simulink model "PSM3_Information_Penkov_Nikolay_Testframework_Gesamtsystem"  (R2012b)
settings: Solver=FixedStepDiscrete  StartTime=0.0  StopTime=320  FixedStep=0.00001  RelTol=1e-3
libraries: idelinklib_tgtpref x1
settings Model: Creator=Nikolay  LastModifiedBy=Nikolay
settings DataIOCC: SaveOutput=off  SaveTime=off
settings OptimizationCC: OptimizeModelRefInitCode=on  LifeSpan=1
settings HardwareCC: ProdBitPerChar=16  ProdBitPerInt=16  ProdBitPerPointer=16  ProdLargestAtomicInteger=Integer  ProdIntDivRoundTo=Zero  ProdEndianess=LittleEndian  ProdWordSize=16  ProdHWDeviceType=Texas Instruments->C2000
settings RTWCC: SystemTargetFile=idelink_ert.tlc  GenerateMakefile=off  TemplateMakefile=none  Description=IDE Link ERT  ProcessScript=idelink_ert_make_rtw_hook
settings CodeAppCC: IgnoreCustomStorageClasses=off

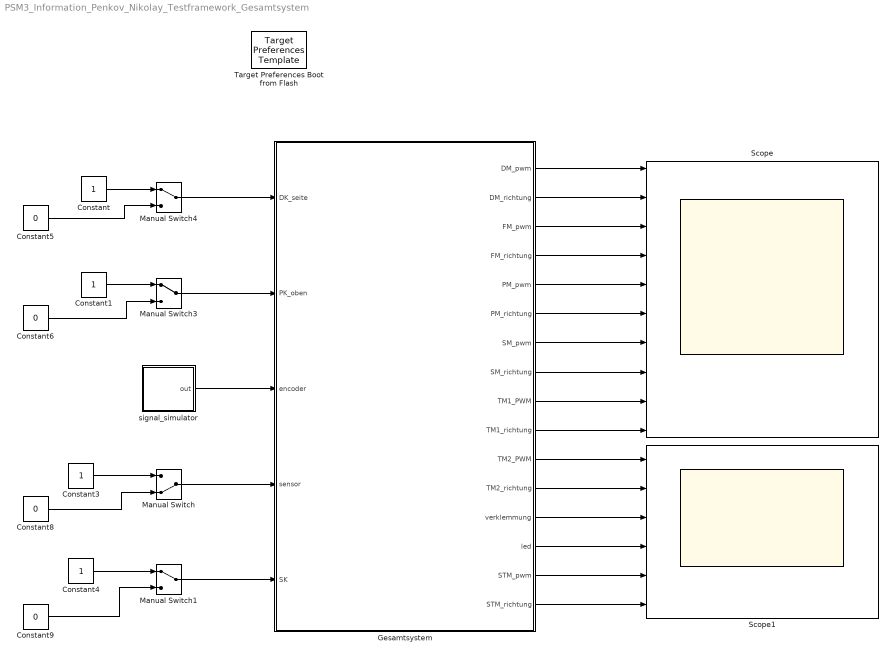
== system PSM3_Information_Penkov_Nikolay_Testframework_Gesamtsystem ==
  Constant{,1,3..4} (4 alike) : Constant
  Constant{5..6,8..9} (4 alike) : Constant  Value=0
  Gesamtsystem : Stateflow chart  TreatAsAtomicUnit=on
  Manual Switch : ManualSwitch  CurrentSetting=0
  Manual Switch1 : ManualSwitch
  Manual Switch3 : ManualSwitch
  Manual Switch4 : ManualSwitch
  Scope : Scope  NumInputPorts=10
      settings: ShowLegends=on  YMin=-1~-1~0~-5~0~-5~-5~-5~-5~-5  YMax=1~1~75~5~100~5~5~5~5~5
  Scope1 : Scope  NumInputPorts=6
      settings: YMin=-5~-5~-5~-5~57~-5  YMax=5~5~5~5~63~5
  Target Preferences Boot from Flash : idelinklib_tgtpref/Target Preferences Template  Tag=ccslinktgtpref_ccsv4  library=off
  signal_simulator : Stateflow chart  TreatAsAtomicUnit=on
  wires:
  signal_simulator/1(out) -> Gesamtsystem/3(encoder)
  Manual Switch1/1 -> Gesamtsystem/5(SK)
  Manual Switch/1 -> Gesamtsystem/4(sensor)
  Manual Switch3/1 -> Gesamtsystem/2(PK_oben)
  Manual Switch4/1 -> Gesamtsystem/1(DK_seite)
  Constant/1 -> Manual Switch4/1
  Constant1/1 -> Manual Switch3/1
  Constant3/1 -> Manual Switch/1
  Constant4/1 -> Manual Switch1/1
  Constant5/1 -> Manual Switch4/2
  Constant6/1 -> Manual Switch3/2
  Constant8/1 -> Manual Switch/2
  Constant9/1 -> Manual Switch1/2
  Gesamtsystem/1(DM_pwm) -> Scope/1
  Gesamtsystem/2(DM_richtung) -> Scope/2
  Gesamtsystem/3(FM_pwm) -> Scope/3
  Gesamtsystem/4(FM_richtung) -> Scope/4
  Gesamtsystem/5(PM_pwm) -> Scope/5
  Gesamtsystem/6(PM_richtung) -> Scope/6
  Gesamtsystem/7(SM_pwm) -> Scope/7
  Gesamtsystem/8(SM_richtung) -> Scope/8
  Gesamtsystem/9(TM1_PWM) -> Scope/9
  Gesamtsystem/10(TM1_richtung) -> Scope/10
  Gesamtsystem/11(TM2_PWM) -> Scope1/1
  Gesamtsystem/12(TM2_richtung) -> Scope1/2
  Gesamtsystem/13(verklemmung) -> Scope1/3
  Gesamtsystem/14(led) -> Scope1/4
  Gesamtsystem/15(STM_pwm) -> Scope1/5
  Gesamtsystem/16(STM_richtung) -> Scope1/6

== stateflow chart PSM3_Information_Penkov_Nikolay_Testframework_Gesamtsystem/Gesamtsystem ==
  state Motor_Foerderbahn_Check [parallel]
    settings: executionOrder=3
    state Start
    state Encoder_abfrage
      zustand_vor = encoder;
    state Naechster_Wert
      zustand_nach = encoder;
    state Vergleich
      vrgl = zustand_nach - zustand_vor;
    state Verklemmt
      verklemmung = true;
    state Nicht_Verklemmt
      verklemmung = false;
    (default) -> Motor_Foerderbahn_Check.Start
    Verklemmt -> Motor_Foerderbahn_Check.Start
    Nicht_Verklemmt -> Motor_Foerderbahn_Check.Start
    Motor_Foerderbahn_Check.Start -> Encoder_abfrage
    Encoder_abfrage -> Naechster_Wert : [after(3,sec)]
    Naechster_Wert -> Vergleich
    Vergleich -> Nicht_Verklemmt [order 2] : [abs(vrgl) == 1]
    Vergleich -> Verklemmt [order 1] : [abs(vrgl) == 0]
  state Teilsystem_1 [parallel]
    settings: executionOrder=1
    state Start
      c = 0;
      turm1_gebaut  = false;
      turm2_gebaut = false;
      led = false;
    state Foerderbahn_start
      en: FM_pwm = 60;
      FM_richtung = 0;
    state System_idle
      FM_pwm = 0;
      TS1_aktivate = false;
      TS2_aktivate = true;
    (default) -> Teilsystem_1.Start
    Teilsystem_1.Start -> Foerderbahn_start
    Teilsystem_1.System_idle -> Foerderbahn_start : [TS1_aktivate == true]
    Foerderbahn_start -> Teilsystem_1.System_idle : [sensor == 0]
  note: INFO: FM_richtung
      | 0 - nach vorne
      | 1 - nach hinten
  state Teilsystem_2 [parallel]
    settings: executionOrder=4
    state TS1_freigabe
      TS2_aktivate = false;
      TS1_aktivate = true;
    state Start
    state Fertig
      led = 1;
    state Platforme_hoch_1
      PM_richtung = 0;
      PM_pwm = 100;
    state System_idle
      TS2_aktivate = false;
      TS3_aktivate = true;
      PM_pwm = 0;
      ex: c = 0;
    state Increment_und_check
      c = c + 1;
    state Plattforme_mittelstop
      PM_pwm = 0;
    state Platforme_runter
      SM_pwm = 0;
      PM_richtung = 1;
      PM_pwm = 100;
    state Stab_entfernen
      STM_richtung = 0;
      STM_pwm = 60;
    state Stab_setzen
      PM_pwm = 0;
      STM_richtung = 1;
      STM_pwm = 60;
    state Platforme_hoch_2
      STM_pwm = 0;
      PM_pwm = 100;
    (default) -> Teilsystem_2.Start
    TS1_freigabe -> Teilsystem_2.Start
    Teilsystem_2.System_idle -> TS1_freigabe [order 1] : [turm2_gebaut == false && TS2_aktivate == true]
    Teilsystem_2.Start -> Platforme_hoch_1 : [TS2_aktivate == true]
    Increment_und_check -> TS1_freigabe [order 2] : [c < 6]
    (junction 437) -> TS1_freigabe [order 2] : [c < 9 && turm1_gebaut == true]
    Teilsystem_2.System_idle -> Fertig [order 2] : [turm2_gebaut == true && TS2_aktivate == true ]
    Platforme_hoch_1 -> Plattforme_mittelstop : after(300,tick)
    (junction 437) -> Teilsystem_2.System_idle [order 1] : [turm1_gebaut == false && c == 6]
    (junction 437) -> Teilsystem_2.System_idle [order 3] : [turm1_gebaut == true && c == 9]
    Increment_und_check -> (junction 437) [order 1] : [c >= 6]
    Plattforme_mittelstop -> Stab_entfernen
    Platforme_runter -> Increment_und_check : after(2,sec)
    Stab_entfernen -> Platforme_hoch_2 : [SK == true]
    Stab_setzen -> Platforme_runter : after(2,sec)
    Platforme_hoch_2 -> Stab_setzen : after(2,sec)
  state Teilsystem_3 [parallel]
    settings: executionOrder=2
    state TS2_freigabe
      TS3_aktivate = false;
      TS2_aktivate = true;
      c =0;
    state Motoren_unter
      TM1_richtung = 1;
      TM2_richtung = 1;
      TM1_PWM = 100;
      TM2_PWM = 100;
      DM_pwm = 0;
    state Start
    state Magazin_transport
      TM1_richtung = 0;
      TM2_richtung = 0;
      TM1_PWM = 100;
      TM2_PWM = 100;
    state Drehen_zureuck
      SM_pwm = 0;
      DM_richtung = 1;
      DM_pwm = 60;
    state Schieber_zureuck
      TM1_PWM = 0;
      TM2_PWM = 0;
      SM_richtung = 1;
      SM_pwm = 60;
    state Hohe_abfrage
      TM1_PWM = 0;
      TM2_PWM = 0;
    state Turm_befreien
      TM1_PWM = 100;
      TM2_PWM = 100;
    state Drehen_T1
      DM_pwm = 60;
      DM_richtung = 0;
      turm1_gebaut = true;
    state Schieber_warten
      SM_pwm = 0;
    state Schieber_fahren
      DM_pwm =0
      SM_richtung = 0;
      SM_pwm = 60;
    state Drehen_T2
      DM_pwm = 60;
      DM_richtung = 0;
      turm2_gebaut = true;
    (default) -> Teilsystem_3.Start
    TS2_freigabe -> Teilsystem_3.Start
    Motoren_unter -> TS2_freigabe : after(3,sec)
    Teilsystem_3.Start -> Magazin_transport : [TS3_aktivate == true]
    Drehen_zureuck -> Motoren_unter : [DK_seite == true]
    Magazin_transport -> Hohe_abfrage : after(3,sec)
    Schieber_zureuck -> Drehen_zureuck : after(1,sec)
    Hohe_abfrage -> (junction 262)
    Turm_befreien -> Schieber_zureuck : after(5,sec)
    Schieber_warten -> Turm_befreien : after(1,sec)
    (junction 262) -> Drehen_T1 [order 1] : [turm1_gebaut == false]
    (junction 262) -> Drehen_T2 [order 2] : [turm1_gebaut == true && turm2_gebaut == false]
    Drehen_T1 -> Schieber_fahren : after(2,sec)
    Schieber_fahren -> Schieber_warten : after(1,sec)
    Drehen_T2 -> Schieber_fahren : after(4,sec)
  note: INFO: PM_richtung
      | 0 - nach oben
      | 1 - nach unten
  note: INFO: TM_richtung
      | 0 - nach oben
      | 1 - nach unten
  note: INFO: STM_richtung
      | 0 - nach hinten
      | 1 - nach vorne
  note: INFO: SM_richtung
      | 0 - nach vorne
      | 1 - nach hinten
  note: INFO: DM_richtung
      | 0 - gegen den Uhrzeigersinn
      | 1 - im Uhrzeigersinn
  data: DK_seite input; PK_oben input; encoder input; sensor input; turm2_gebaut local double; DM_pwm output double; DM_richtung output double; FM_pwm output double; FM_richtung output double; PM_pwm output double; PM_richtung output double; SM_pwm output double; SM_richtung output double; TM1_PWM output double; TM1_richtung output double; TM2_PWM output double; TM2_richtung output double; verklemmung output double; TS1_aktivate local double; TS2_aktivate local double; TS3_aktivate local double; turm1_gebaut local double; vrgl local double; zustand_nach local double; zustand_vor local double; c local double [0..1000] =0; led output double; STM_pwm output double; STM_richtung output double; SK input

== stateflow chart PSM3_Information_Penkov_Nikolay_Testframework_Gesamtsystem/signal_simulator ==
  state Signal_on
    out = 1;
  state Signal_off
    out = 0;
  (default) -> Signal_on
  Signal_on -> Signal_off : after(1,sec)
  Signal_off -> Signal_on : after(1,sec)
  data: out output double
